simulink model "SiEngineCore"  (R2018a)
settings: Solver=VariableStepAuto  StartTime=0.0  StopTime=inf  RelTol=1e-3  EnableMultiTasking=on
model workspace (MAT data in the model file):
  AFRStoich = 14.6
  AirFilterArea = 0.000962112750162
  AirIntakeVol = 0.0137
  C_eng = 40000
  CompEff = [0.2 0.2 0.2 0.2 0.2 0.2 0.2 0.2 0.2 0.2 0.2 0.2 ... (5000 elements, 50x100)]
  CompMassFlwRate = [4.4091251837e-05 0.00441685548409 0.00879200250921 0.0131688186568 0.0175465480563 0.0219243905675 0.0263014996182 0.0306769799437 0.0350498852261 0.0394192156283 0.0437839152204 0.0481428692931 ... (5000 elements, 50x100)]
  CompPrsRatioBreakPoints = [1 1.02808080808 1.05616161616 1.08424242424 1.11232323232 1.1404040404 1.16848484848 1.19656565657 1.22464646465 1.25272727273 1.28080808081 1.30888888889 1.33696969697 1.36505050505 1.39313131313 1.42121212121 1.44929292929 1.47737373737 1.50545454545 1.53353535354 1.56161616162 1.5896969697 1.61777777778 1.64585858586 1.67393939394 1.70202020202 1.7301010101 1.75818181818 1.78626262626 1.81434343434 1.84242424242 1.87050505051 1.89858585859 1.92666666667 1.95474747475 1.98282828283 2.01090909091 2.03898989899 2.06707070707 2.09515151515 2.12323232323 2.15131313131 2.17939393939 2.20747474747 2.23555555556 2.26363636364 2.29171717172 2.3197979798 2.34787878788 2.37595959596 2.40404040404 2.43212121212 2.4602020202 2.48828282828 2.51636363636 2.54444444444 2.57252525253 2.60060606061 2.62868686869 2.65676767677 2.68484848485 2.71292929293 2.74101010101 2.76909090909 2.79717171717 2.82525252525 2.85333333333 2.88141414141 2.90949494949 2.93757575758 2.96565656566 2.99373737374 3.02181818182 3.0498989899 3.07797979798 3.10606060606 3.13414141414 3.16222222222 3.1903030303 3.21838383838 3.24646464646 3.27454545455 3.30262626263 3.33070707071 3.35878787879 3.38686868687 3.41494949495 3.44303030303 3.47111111111 3.49919191919 3.52727272727 3.55535353535 3.58343434343 3.61151515152 3.6395959596 3.66767676768 3.69575757576 3.72383838384 3.75191919192 3.78]
  CompRefPrs = 101325
  CompRefTemp = 300
  CompSpdBreakPoints = [5 500.713942607 996.427885215 1492.14182782 1987.85577043 2483.56971304 2979.28365564 3474.99759825 3970.71154086 4466.42548347 4962.13942607 5457.85336868 5953.56731129 6449.2812539 6944.9951965 7440.70913911 7936.42308172 8432.13702433 8927.85096693 9423.56490954 9919.27885215 10414.9927948 10910.7067374 11406.42068 11902.1346226 12397.8485652 12893.5625078 13389.2764504 13884.990393 14380.7043356 14876.4182782 15372.1322208 15867.8461634 16363.560106 16859.2740487 17354.9879913 17850.7019339 18346.4158765 18842.1298191 19337.8437617 19833.5577043 20329.2716469 20824.9855895 21320.6995321 21816.4134747 22312.1274173 22807.8413599 23303.5553025 23799.2692452 24294.9831878]
  CoolantTemp = 310
  Cps = 2
  EgrArea = 0.000314159265359
  EgrCoolantTemp = 360
  EgrEffectiveness = 0.8
  ExhSysArea = 0.00138544236023
  ExhSysVol = 0.0044
  IcEffectiveness = 0.7
  InjSlp = 6.45161290323
  LHV = 47300000
  NCyl = 4
  Pstd = 101325
  Rair = 287
  Rexh = 297
  T_cool_start = 355
  T_coolnt_init = 355
  T_coolnt_max = 375
  ThrAngToC = [0  0.001; 90  0.735]
  ThrDiam = 50
  Tstd = 293.15
  TurbEff = [0.1 0.1 0.1 0.1 0.1 0.1 0.1 0.1 0.1 0.1 0.1 0.1 ... (3600 elements, 60x60)]
  TurbMassFlwRate = [0 0 0 0 0 0 0 0 0 0 0 0 ... (3600 elements, 60x60)]
  TurbPrsRatioBreakPoints = [1 1.0066198 1.0187236 1.0343974 1.0529583 1.0740113 1.0972904 1.1226 1.1497884 1.178734 1.2093357 1.2415084 1.2751789 1.3102832 1.346765 1.3845742 1.4236656 1.4639986 1.5055358 1.5482436 1.5920907 1.637048 1.6830889 1.7301885 1.7783234 1.8274719 1.8776134 1.9287287 1.9807996 2.0338087 2.08774 2.142578 2.1983073 2.2549145 2.312386 2.3707092 2.4298713 2.4898612 2.5506673 2.6122787 2.6746855 2.737877 2.801844 2.8665771 2.9320674 2.998306 3.065285 3.1329958 3.201431 3.270583 3.3404438 3.4110072 3.4822657 3.5542126 3.6268415 3.7001462 3.7741203 3.8487577 3.924053 4]
  TurbRefPres = 101325
  TurbRefTemp = 300
  TurbSpdBreakPoints = [0; 236.716179913; 473.432359826; 710.148557878; 946.864755929; 1183.5809177; 1420.29711576; 1657.01327753; 1893.72933048; 2130.44574618; 2367.16179913; 2603.87821484; 2840.59426779; 3077.31050211; 3314.02673644; 3550.74278939; 3787.45884233; 4024.17507666; 4260.89149237; 4497.6077267; 4734.32359826; 4971.04001397; 5207.7562483; 5444.47211987; 5681.18853557; 5917.90495128; 6154.62118561; 6391.33705717; 6628.0532915; 6864.76952583; 7101.48557878; 7338.2018131; 7574.91768467; 7811.6348259; 8048.35015332; 8285.06620627; 8521.78262198; 8758.49885631; 8995.21563477; 9231.93150634; 9468.64755929; 9705.36415637; 9942.08002794; 10178.7958995; 10415.5124966; 10652.2283682; 10888.9442397; 11125.6610182; 11362.3768898; 11599.0927613; 11835.8099026; 12072.52523; 12309.2423712; 12545.9576986; 12782.673933; 13019.3907114; 13256.106583; 13492.8226359; 13729.539233; 13966.2551046]
  TurboInertia = 1.55e-05
  Vd = 0.0015
  Vexh = 0.0016
  Vint = 0.00286
  VolCompOut = 0.0026
  WgArea = 0.000314159265359
  cp_air = 1005
  cp_exh = 1005
  f_co = [6.86026635502e-05 6.86026635502e-05 0.000137130178455 0.000177313004818 0.000153545722458 0.000286109103754 0.00065603982686 0.00012726330728 0.000129286672759 0.000129286672759 0.000129286672759 0.000129286672759 ... (240 elements, 16x15)]
  f_co2 = [0.190124640361 0.190124640361 0.197310430134 0.198841052192 0.19976911847 0.200569885042 0.199664821109 0.20034918367 0.20035007673 0.20035007673 0.20035007673 0.20035007673 ... (240 elements, 16x15)]
  f_del_sa_bpt = [0 0.75 1.5 2.25 3 3.75 4.5 5.25 6 6.75 7.5 8.25 9 9.75 10.5 11.25 12 12.75 13.5 14.25 15 15.75 16.5 17.25 18 18.75 19.5 20.25 21 21.75 22.5 23.25 24 24.75 25.5 26.25 27 27.75 28.5 29.25 30 30.75 31.5 32.25 33 33.75 34.5 35.25 36 36.75 37.5 38.25 39 39.75 40.5 41.25 42 42.75 43.5 44.25 45 45.75 46.5 47.25 48]
  f_exhfrac_n_bpt = [750 1053.57142857 1357.14285714 1660.71428571 1964.28571429 2267.85714286 2571.42857143 2875 3178.57142857 3482.14285714 3785.71428571 4089.28571429 4392.85714286 4696.42857143 5000]
  f_exhfrac_trq_bpt = [0 15 26.4285714286 37.8571428571 49.2857142857 60.7142857143 72.1428571429 83.5714285714 95 106.428571429 117.857142857 129.285714286 140.714285714 152.142857143 163.571428571 175]
  f_fric_temp_bpt = [274 276 278 280 282 284 286 288 290 292 294 296 298 300 302 304 306 308 310 312 314 316 318 320 322 324 326 328 330 332 334 336 338 340 342 344 346 348 350 352 354 356 358 360 362 364 366 368 370 372 374 376 378 380]
  f_fric_temp_mod = [3.96 3.22 2.56 2.26 2.11 2 1.9 1.83 1.76 1.7 1.65 1.6 1.55 1.49 1.44 1.41 1.38 1.35 1.32 1.3 1.27 1.25 1.24 1.21 1.2 1.18 1.16 1.15 1.13 1.12 1.11 1.1 1.09 1.08 1.07 1.06 1.05 1.05 1.04 1.03 1.02 1.02 1.01 1.01 1 1 1 0.999 0.997 0.995 0.993 0.991 0.989 0.987]
  f_hc = [0.00443209119576 0.00443209119576 0.00220684816441 0.00166684424867 0.00138421884093 0.0010658858934 0.00112857643245 0.00117703080332 0.00117597584116 0.00117597584116 0.00117597584116 0.00117597584116 ... (240 elements, 16x15)]
  f_m_lam = [0.94128 0.95565 0.97001 0.98437 0.99008 1.0004 0.97527 0.9549 0.92612 0.89735 0]
  f_m_lam_bpt = [0.65 0.7 0.75 0.8 0.85 0.9 0.95 1 1.05 1.1 2]
  f_m_sa = [1.0019 0.9988 0.9953 0.99173 0.98811 0.98441 0.98065 0.97682 0.97293 0.96897 0.96493 0.96083 0.95666 0.95242 0.94811 0.94373 0.93927 0.93475 0.93015 0.92548 0.92074 0.91592 0.91104 0.90608 0.90105 0.89594 0.89076 0.88551 0.88019 0.8748 0.86933 0.86379 0.85818 0.8525 0.84675 0.84093 0.83503 0.82907 0.82303 0.81693 0.81075 0.80451 0.79819 0.79181 0.78536 0.77884 0.77226 0.7656 0.75888 0.75209 0.74524 0.73832 0.73134 0.72429 0.71717 0.70999 0.70275 0.69682 0.68949 0.68303 0.67548 0.67037 0.66525 0.66014 0.65503]
  f_mdot_air_corr = [1.02156051768 1.00597426471 0.989411677851 1.0033499089 0.984591437857 0.988509040623 1.0326198627 1.02765527362 1.0134784519 0.998280021213 0.981755128787 0.967218261288 ... (400 elements, 20x20)]
  f_mdot_air_corr_ld_bpt = [0.223381333333 0.285105122807 0.346828912281 0.408552701754 0.470276491228 0.532000280702 0.593724070175 0.655447859649 0.717171649123 0.778895438596 0.84061922807 0.902343017544 0.964066807018 1.02579059649 1.08751438596 1.14923817544 1.21096196491 1.27268575439 1.33440954386 1.39613333333]
  f_mdot_air_n_bpt = [750 973.6842 1197.3684 1421.0526 1644.7368 1868.4211 2092.1053 2315.7895 2539.4737 2763.1579 2986.8421 3210.5263 3434.2105 3657.8947 3881.5789 4105.2632 4328.9474 4552.6316 4776.3158 5000]
  f_mdot_intk = [0 0 0 0 0 0 0 0 0 0 0 0 ... (400 elements, 20x20)]
  f_mdot_intk_ecp_bpt = [0 2.6316 5.2632 7.8947 10.5263 13.1579 15.7895 18.4211 21.0526 23.6842 26.3158 28.9474 31.5789 34.2105 36.8421 39.4737 42.1053 44.7368 47.3684 50]
  f_mdot_trpd_bpt = [0 5.7895 11.5789 17.3684 23.1579 28.9474 34.7368 40.5263 46.3158 52.1053 57.8947 63.6842 69.4737 75.2632 81.0526 86.8421 92.6316 98.4211 104.2105 110]
  f_nox = [4.08881357131e-05 4.08881357131e-05 0.00012346903723 0.000189339284589 0.00026637780763 0.000608287545555 0.00102018770254 0.00131576653087 0.00131610412986 0.00131610412986 0.00131610412986 0.00131610412986 ... (240 elements, 16x15)]
  f_nv = [0.64175366561 0.641419295169 0.640125365558 0.638690556197 0.644169906538 0.669178791311 0.731659452876 0.750078238889 0.750078238889 0.750078238889 0.750078238889 0.750078238889 ... (225 elements, 15x15)]
  f_nv_n_bpt = [750 1053.57142857 1357.14285714 1660.71428571 1964.28571429 2267.85714286 2571.42857143 2875 3178.57142857 3482.14285714 3785.71428571 4089.28571429 4392.85714286 4696.42857143 5000]
  f_nv_prs_bpt = [31 40.6428571429 50.2857142857 59.9285714286 69.5714285714 79.2142857143 88.8571428571 98.5 108.142857143 117.785714286 127.428571429 137.071428571 146.714285714 156.357142857 166]
  f_sa_opt = [35.3085 35.3085 21.0105 10.3714 8.5076 7.1426 7.5656 -5.7766 -16.7061 -16.8345 -19.3546 -20.6085 ... (256 elements, 16x16)]
  f_t_exh = [739.936218766 750.584766028 772.770773797 791.235245621 803.106549716 885.862998064 920.498479307 920.498479307 920.498479307 920.498479307 920.498479307 920.498479307 ... (225 elements, 15x15)]
  f_t_exh_l_bpt = [0.2 0.275 0.35 0.425 0.5 0.575 0.65 0.725 0.8 0.875 0.95 1.025 1.1 1.175 1.25]
  f_t_exh_n_bpt = [750 1053.57142857 1357.14285714 1660.71428571 1964.28571429 2267.85714286 2571.42857143 2875 3178.57142857 3482.14285714 3785.71428571 4089.28571429 4392.85714286 4696.42857143 5000]
  f_tm_corr = [0.839360054391 0.833393271885 0.82629554201 0.818442814437 0.811524387436 0.809164184856 0.814606352881 0.826887956871 0.842304598924 0.856886829014 0.869487025783 0.880530414174 ... (400 elements, 20x20)]
  f_tm_corr_n_bpt = [750 973.6842 1197.3684 1421.0526 1644.7368 1868.4211 2092.1053 2315.7895 2539.4737 2763.1579 2986.8421 3210.5263 3434.2105 3657.8947 3881.5789 4105.2632 4328.9474 4552.6316 4776.3158 5000]
  f_tm_corr_nd_bpt = [0.3 0.38947 0.47895 0.56842 0.65789 0.74737 0.83684 0.92632 1.0158 1.1053 1.1947 1.2842 1.3737 1.4632 1.5526 1.6421 1.7316 1.8211 1.9105 2]
  f_tq_fric = [0  4.16  4.8  5.44  6.05  6.64  7.23  7.81  8.39  8.97  9.54  10.1  10.7  11.3  11.9  12.5; 0  4.16  4.8  5.44  6.05  6.64  7.23  7.81  8.39  8.97  9.54  10.1  10.7  11.3  11.9  12.5; 0  4.42  5.07  5.69  6.29  6.89  7.49  8.09  8.69  9.28  9.86  10.4  11  11.6  12.2  12.8; 0  4.69  5.36  5.98  6.58  7.18  7.79  8.41  9.02  9.62  10.2  10.8  11.4  11.9  12.5  13.1; 0  4.88  5.59  6.25  6.87  7.48  8.09  8.71  9.32  9.92  10.5  11.1  11.7  12.3  12.9  13.4; 0  4.94  5.74  6.45  7.12  7.75  8.37  8.99  9.59  10.2  10.8  11.4  11.9  12.6  13.2  13.8; 0  4.93  5.76  6.56  7.29  7.97  8.62  9.23  9.83  10.4  11  11.6  12.2  12.8  13.4  14.1; 0  4.85  5.67  6.57  7.37  8.11  8.8  9.43  10  10.6  11.2  11.8  12.4  13  13.7  14.3; 0  4.74  5.57  6.46  7.34  8.14  8.88  9.55  10.2  10.8  11.4  12  12.6  13.2  13.8  14.4; 0  4.63  5.42  6.27  7.19  8.05  8.83  9.55  10.2  10.9  11.5  12.1  12.7  13.3  14  14.6; 0  4.52  5.29  6.11  6.98  7.84  8.65  9.4  10.1  10.8  11.5  12.1  12.8  13.4  14.1  14.6; 0  4.42  5.18  5.97  6.79  7.6  8.39  9.15  9.88  10.6  11.3  12.1  12.8  13.5  14.1  14.7; 0  4.34  5.09  5.86  6.64  7.42  8.17  8.88  9.6  10.3  11.1  11.9  12.7  13.4  14.1  14.7; 0  4.27  5.01  5.76  6.52  7.28  8.03  8.74  9.39  10.1  10.8  11.6  12.4  13.2  14  14.7; 0  4.21  4.94  5.67  6.42  7.16  7.89  8.59  9.25  9.93  10.7  11.5  12.3  13.1  13.8  14.6; 0  4.15  4.87  5.6  6.33  7.06  7.77  8.47  9.14  9.84  10.6  11.3  12.1  12.9  13.7  14.4]
  f_tq_inr = [25.8508 25.8508 25.8508 25.8508 25.8508 25.8508 25.8508 25.8508 25.8508 25.8508 25.8508 25.8508 ... (256 elements, 16x16)]
  f_tq_inr_l_bpt = [0.1 0.2 0.28571 0.37143 0.45714 0.54286 0.62857 0.71429 0.8 0.88571 0.97143 1.0571 1.1429 1.2286 1.3143 1.4]
  f_tq_inr_n_bpt = [0 750 1053.5714 1357.1429 1660.7143 1964.2857 2267.8571 2571.4286 2875 3178.5714 3482.1429 3785.7143 4089.2857 4392.8571 4696.4286 5000]
  f_tq_nl = [0 15.0012133443 26.4298333923 37.8556656512 49.2846782956 60.7113978793 72.3451969202 77.459652163 78.5324534074 78.5324534074 78.5324534074 78.5324534074 ... (256 elements, 16x16)]
  f_tq_nl_l_bpt = [0 0.2 0.275 0.35 0.425 0.5 0.575 0.65 0.725 0.8 0.875 0.95 1.025 1.1 1.175 1.25]
  f_tq_nl_n_bpt = [0 750 1053.57142857 1357.14285714 1660.71428571 1964.28571429 2267.85714286 2571.42857143 2875 3178.57142857 3482.14285714 3785.71428571 4089.28571429 4392.85714286 4696.42857143 5000]
  f_tq_pump = [0  7.24  7.7  7.82  7.95  8.1  8.27  8.45  8.64  8.78  8.88  8.96  9.03  9.12  9.25  9.45; 0  7.24  7.7  7.82  7.95  8.1  8.27  8.45  8.64  8.78  8.88  8.96  9.03  9.12  9.25  9.45; 0  5.67  6.03  6.37  6.67  6.92  7.14  7.33  7.5  7.67  7.84  8.01  8.19  8.38  8.58  8.8; 0  3.94  4.52  5  5.36  5.6  5.77  5.92  6.1  6.35  6.67  7.02  7.4  7.75  8.06  8.34; 0  2.59  3.14  3.57  3.86  4.05  4.21  4.43  4.76  5.21  5.75  6.32  6.85  7.3  7.65  7.92; 0  1.8  2.25  2.61  2.88  3.11  3.37  3.71  4.17  4.74  5.36  5.96  6.49  6.91  7.23  7.46; 0  1  1.36  1.77  2.15  2.51  2.88  3.31  3.8  4.37  4.98  5.57  6.11  6.57  6.94  7.25; 0  1  1  1  1.09  1.59  2.08  2.6  3.17  3.81  4.49  5.19  5.85  6.44  6.92  7.29; 0  1  1  1  1  1  1.62  2.32  3.05  3.83  4.64  5.44  6.19  6.82  7.31  7.65; 0  1  1  1  1  1  1.35  2.21  3.08  3.97  4.88  5.78  6.64  7.41  8.06  8.58; 0  1  1  1  1  1  1  1.77  2.67  3.58  4.55  5.6  6.73  7.91  9.07  10.1; 0  1  1  1  1  1  1  1.72  2.67  3.61  4.62  5.79  7.15  8.69  10.3  11.9; 0  1  1  1  1  1  1  1.74  2.88  3.96  5.08  6.36  7.86  9.57  11.4  13.2; 0  1  1  1  1  1  1  1.37  2.7  4.01  5.39  6.92  8.65  10.5  12.4  14.2; 0  1  1  1  1  1  1  1.28  2.66  4.14  5.72  7.43  9.28  11.2  13.1  14.8; 0  1  1  1  1  1  1  1.39  2.82  4.39  6.06  7.85  9.73  11.6  13.5  15.1]
  f_vivc = [0.37716 0.38164 0.38611 0.39033 0.39428 0.39795 0.40132 0.40441 0.40719 0.40967 0.41184 0.41372 0.41529 0.41656 0.41755 0.41825 0.41867 0.41884 0.41874 0.41865]
  f_vivc_icp_bpt = [0 2.6316 5.2632 7.8947 10.5263 13.1579 15.7895 18.4211 21.0526 23.6842 26.3158 28.9474 31.5789 34.2105 36.8421 39.4737 42.1053 44.7368 47.3684 50]
  tau_cool = 3000
libraries: autolibfundflw x13, autolibboost x3, simulink x1, autolibcoreeng x1
(part 1 of 2)
settings Model: ModifiedByFormat=The MathWorks, Inc.  Creator=The MathWorks, Inc.  LastModifiedBy=The MathWorks, Inc.
settings DataIOCC: DSMLogging=off
settings CodeAppCC: StateflowObjectComments=on
settings GRTTargetCC: TargetLangStandard=C89/C90 (ANSI)
settings ConfigComp: CovMetricSettings=dsw  CovHtmlReporting=on  CovSaveCumulativeToWorkspaceVar=on  CovSaveSingleToWorkspaceVar=on  CovShowResultsExplorer=off  CovExternalEMLEnable=off
settings SimscapeCC: SimscapeNormalizeSystem=off  SimscapeNominalValues={1, 'bar'; 1, 'cm^3/s'; 1, 'bar*kg/s'; 1, 'kJ/kg'; 1, 'kW'; }

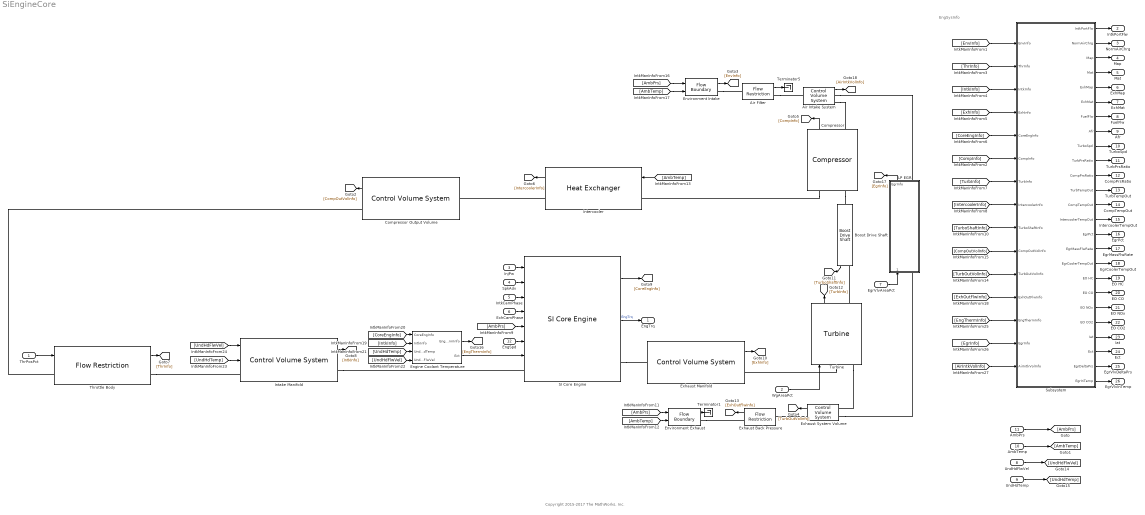
== system SiEngineCore ==
  note: EngSysInfo
  note: Copyright 2015-2017 The MathWorks, Inc.
  ThrPosPct : Inport
  WgAreaPct : Inport  Port=2
  InjPw : Inport  Port=3
  SpkAdv : Inport  Port=4
  IntkCamPhase : Inport  Port=5
  ExhCamPhase : Inport  Port=6
  EgrVlvAreaPct : Inport  Port=7
  UndHdFlwVel : Inport  Port=8
  UndHdTemp : Inport  Port=9
  AmbTemp : Inport  Port=10
  AmbPrs : Inport  Port=11
  EngSpd : Inport  Port=12
  Air Filter : autolibfundflw/Flow Restriction  AreaPopup=Constant  ImageTypePopup=Cold  gamma=cp_air/(cp_air-Rair)  R=Rair  Plim=0.9  Aorf_cnst=AirFilterArea  Cd_cnst=1  Cd_ext=1  Dthr=50  ThrCd=[0.001; 0.735]  ThrAngBpts=[0; 90]
      settings: SourceProductName=Powertrain Blockset  SourceProductBaseCode=PW
  Air Intake System : autolibfundflw/Control Volume System  NumInletPorts=1  NumOutletPorts=2  HeatTransferModelPopup=Constant  ImageTypePopup=Cold  Vch=AirIntakeVol  Pinit=101325  Tinit=298  R=Rair  cp=cp_air  q_he=0  ext_tbl=[40 160 740 2000]  ext_bpts=linspace(0,180,4)  Aext_conv=0.125  m_wall=7  cp_wall=900  Tmass=293.15  Dext_cond=0.004  Aext_cond=0.003  kext=25  Dint_cond=0.004  Aint_cond=0.003  kint=25  int_tbl=[40 160 740 2000]  int_bpts=linspace(0.0020,0.1100,4)  Aint_conv=0.125
      settings: SourceProductName=Powertrain Blockset  SourceProductBaseCode=PW
  Boost Drive Shaft : autolibboost/Boost Drive Shaft  ShaftConfigPopup=Turbocharger  AddTrqTypePopup=No external torque  J_shaft=TurboInertia  w_0=5000*pi/30  w_min=1  w_max=1e6  eta_mech=1
      settings: SourceProductName=Powertrain Blockset  SourceProductBaseCode=PW
  Compressor : autolibboost/Compressor  mdot_corr_tbl=CompMassFlwRate  eta_comp_tbl=CompEff  w_corr_bpts1=CompSpdBreakPoints  Pr_bpts2=CompPrsRatioBreakPoints  T_ref=CompRefTemp  P_ref=CompRefPrs  R=Rair  cp=cp_air
      settings: SourceProductName=Powertrain Blockset  SourceProductBaseCode=PW
  Compressor Output Volume : autolibfundflw/Control Volume System  NumInletPorts=1  NumOutletPorts=1  HeatTransferModelPopup=Constant  ImageTypePopup=Cold  Vch=VolCompOut  Pinit=101325  Tinit=298  R=Rair  cp=cp_air  q_he=0  ext_tbl=[40 160 740 2000]  ext_bpts=linspace(0,180,4)  Aext_conv=0.125  m_wall=7  cp_wall=900  Tmass=293.15  Dext_cond=0.004  Aext_cond=0.003  kext=25  Dint_cond=0.004  Aint_cond=0.003  kint=25  int_tbl=[40 160 740 2000]  int_bpts=linspace(0.0020,0.1100,4)  Aint_conv=0.125
      settings: SourceProductName=Powertrain Blockset  SourceProductBaseCode=PW
  Engine Coolant Temperature : Subsystem
  Environment Exhaust : autolibfundflw/Flow Boundary  PrsTempSrcPopup=External input  ImageTypePopup=Hot  Pcnst=101325  Tcnst=298.15  cp=cp_air
      settings: SourceProductName=Powertrain Blockset  SourceProductBaseCode=PW
  Environment Intake : autolibfundflw/Flow Boundary  PrsTempSrcPopup=External input  ImageTypePopup=Cold  Pcnst=101325  Tcnst=298.15  cp=cp_air
      settings: SourceProductName=Powertrain Blockset  SourceProductBaseCode=PW
  Exhaust Back Pressure : autolibfundflw/Flow Restriction  AreaPopup=Constant  ImageTypePopup=Hot  gamma=cp_exh/(cp_exh-Rexh)  R=Rexh  Plim=0.9  Aorf_cnst=ExhSysArea  Cd_cnst=1  Cd_ext=1  Dthr=50  ThrCd=[0.001; 0.735]  ThrAngBpts=[0; 90]
      settings: SourceProductName=Powertrain Blockset  SourceProductBaseCode=PW
  Exhaust Manifold : autolibfundflw/Control Volume System  NumInletPorts=1  NumOutletPorts=1  HeatTransferModelPopup=Constant  ImageTypePopup=Hot  Vch=Vexh  Pinit=101325  Tinit=298  R=Rexh  cp=cp_exh  q_he=0  ext_tbl=[40 160 740 2000]  ext_bpts=linspace(0,180,4)  Aext_conv=0.125  m_wall=7  cp_wall=900  Tmass=293.15  Dext_cond=0.004  Aext_cond=0.003  kext=25  Dint_cond=0.004  Aint_cond=0.003  kint=25  int_tbl=[40 160 740 2000]  int_bpts=linspace(0.0020,0.1100,4)  Aint_conv=0.125
      settings: SourceProductName=Powertrain Blockset  SourceProductBaseCode=PW
  Exhaust System Volume : autolibfundflw/Control Volume System  NumInletPorts=2  NumOutletPorts=1  HeatTransferModelPopup=Constant  ImageTypePopup=Hot  Vch=ExhSysVol  Pinit=101325  Tinit=298  R=Rexh  cp=cp_exh  q_he=0  ext_tbl=[40 160 740 2000]  ext_bpts=linspace(0,180,4)  Aext_conv=0.125  m_wall=7  cp_wall=900  Tmass=293.15  Dext_cond=0.004  Aext_cond=0.003  kext=25  Dint_cond=0.004  Aint_cond=0.003  kint=25  int_tbl=[40 160 740 2000]  int_bpts=linspace(0.0020,0.1100,4)  Aint_conv=0.125
      settings: SourceProductName=Powertrain Blockset  SourceProductBaseCode=PW
  Intake Manifold : autolibfundflw/Control Volume System  NumInletPorts=1  NumOutletPorts=1  HeatTransferModelPopup=External wall convection  ImageTypePopup=Cold  Vch=Vint  Pinit=101325  Tinit=298  R=Rair  cp=cp_air  q_he=0  ext_tbl=[40 160 740 2000]  ext_bpts=linspace(0,180,4)  Aext_conv=0.125  m_wall=7  cp_wall=900  Tmass=293.15  Dext_cond=0.004  Aext_cond=0.003  kext=25  Dint_cond=0.004  Aint_cond=0.003  kint=25  int_tbl=[40 160 740 2000]  int_bpts=linspace(0.0020,0.1100,4)  Aint_conv=0.125
      settings: SourceProductName=Powertrain Blockset  SourceProductBaseCode=PW
  Intercooler : autolibfundflw/Heat Exchanger  EffctModelPopup=Constant  CoolTempInputPopup=External input  ImageTypePopup=Intercooler  ep_cnst=IcEffectiveness  T_cool_cnst=CoolantTemp  cp=cp_air
      settings: SourceProductName=Powertrain Blockset  SourceProductBaseCode=PW
  LP EGR : Subsystem
  SI Core Engine : autolibcoreeng/SI Core Engine  AirMassFlowOptionPopup=Dual-Independent Variable Cam Phasing  TrqOptionPopup=Torque Structure  NCyl=NCyl  Cps=Cps  Vd=Vd  Rair=Rair  Pstd=Pstd  Tstd=Tstd  f_nv=f_nv  f_nv_prs_bpt=f_nv_prs_bpt  f_nv_n_bpt=f_nv_n_bpt  f_vivc=f_vivc  f_vivc_icp_bpt=f_vivc_icp_bpt  f_tm_corr=f_tm_corr  f_tm_corr_nd_bpt=f_tm_corr_nd_bpt  f_tm_corr_n_bpt=f_tm_corr_n_bpt  f_mdot_intk=f_mdot_intk  f_mdot_intk_ecp_bpt=f_mdot_intk_ecp_bpt  f_mdot_trpd_bpt=f_mdot_trpd_bpt  f_mdot_air_corr=f_mdot_air_corr  f_mdot_air_corr_ld_bpt=f_mdot_air_corr_ld_bpt  f_mdot_air_n_bpt=f_mdot_air_n_bpt  f_tq_nl=f_tq_nl  f_tq_nl_l_bpt=f_tq_nl_l_bpt  f_tq_nl_n_bpt=f_tq_nl_n_bpt  f_tq_inr=f_tq_inr  f_tq_fric=f_tq_fric  f_fric_temp_mod=f_fric_temp_mod  f_fric_temp_bpt=f_fric_temp_bpt  f_tq_pump=f_tq_pump  f_sa_opt=f_sa_opt  f_tq_inr_l_bpt=f_tq_inr_l_bpt  f_tq_inr_n_bpt=f_tq_inr_n_bpt  f_m_sa=f_m_sa  f_del_sa_bpt=f_del_sa_bpt  f_m_lam=f_m_lam  f_m_lam_bpt=f_m_lam_bpt  f_t_exh=f_t_exh  f_t_exh_l_bpt=f_t_exh_l_bpt  f_t_exh_n_bpt=f_t_exh_n_bpt  cp_exh=cp_exh  CO2EmissionsCheckbox=on  COEmissionsCheckbox=on  NOxEmissionsCheckbox=on  HCEmissionsCheckbox=on  PMEmissionsCheckbox=off  f_CO2_frac=f_co2  f_CO_frac=f_co  f_HC_frac=f_hc  f_NOx_frac=f_nox  f_PM_frac=[0 0 0 0 0 0 0 0 0 0 0 0 0 0 0;0 0 0 0 0 0 0 0 0 0 0 0 0 0 0;0 0 0 0 0 0 0 0 0 0 0 0 0 0 0;0 0 0 0 0 0 0 0 0 0 0 0 0 0 0;0 0 0 0 0 0 0 0 0 0 0 0 0 0 0;0 0 0 0 0 0 0 0 0 0 0 0 0 0 0;0 0 0 0 0 0 0 0 0 0 0 0 0 0 0;0 0 0 0 0 0 0 0 0 0 0 0 0 0 0;0 0 0 0 0 0 0 0 0 0 0 0 0 0 0;0 0 0 0 0 0 0 0 0 0 0 0 0 0 0;0 0 0 0 0 0 0 0 0 0 0 0 0 0 0;0 0 0 0 0 0 0 0 0 0 0 0 0 0 0;0 0 0 0 0 0 0 0 0 0 0 0 0 0 0;0 0 0 0 0 0 0 0 0 0 0 0 0 0 0;0 0 0 0 0 0 0 0 0 0 0 0 0 0 0;0 0 0 0 0 0 0 0 0 0 0 0 0 0 0]  f_exhfrac_n_bpt=f_exhfrac_n_bpt  f_exhfrac_trq_bpt=f_exhfrac_trq_bpt  Sinj=InjSlp  afr_stoich=AFRStoich
      settings: SourceProductName=Powertrain Blockset  SourceProductBaseCode=PW
  Subsystem : Subsystem
  Terminator1 : Terminator
  Terminator5 : Terminator
  Throttle Body : autolibfundflw/Flow Restriction  AreaPopup=Throttle body geometry  ImageTypePopup=Cold  gamma=cp_air / (cp_air - Rair)  R=Rair  Plim=0.9  Aorf_cnst=.1  Cd_cnst=1  Cd_ext=1  Dthr=ThrDiam  ThrCd=ThrAngToC(:,2)  ThrAngBpts=ThrAngToC(:,1)
      settings: SourceProductName=Powertrain Blockset  SourceProductBaseCode=PW
  Turbine : autolibboost/Turbine  TurbTypePopup=Fixed geometry  WgIncludeCheckbox=on  mdot_corrfx_tbl=TurbMassFlwRate  mdot_corrvr_tbl=TurbMassFlwRate  eta_turbfx_tbl=TurbEff  eta_turbvr_tbl=TurbEff  w_corrfx_bpts1=TurbSpdBreakPoints  w_corrvr_bpts2=TurbSpdBreakPoints  Pr_fx_bpts2=TurbPrsRatioBreakPoints  Pr_vr_bpts2=TurbPrsRatioBreakPoints  L_rack_bpts3=TurbRackBreakPoints  T_ref=TurbRefTemp  P_ref=TurbRefPres  mdot_thresh=1e-6  A_wgopen=WgArea  Plim_wg=0.95  R=Rexh  cp=cp_exh
      settings: SourceProductName=Powertrain Blockset  SourceProductBaseCode=PW
  EngTrq : Outport
  IntkPortFlw : Outport  Port=2
  NormAirChrg : Outport  Port=3
  Map : Outport  Port=4
  Mat : Outport  Port=5
  ExhMap : Outport  Port=6
  ExhMat : Outport  Port=7
  FuelFlw : Outport  Port=8
  Afr : Outport  Port=9
  TurboSpd : Outport  Port=10
  TurbPrsRatio : Outport  Port=11
  CompPrsRatio : Outport  Port=12
  TurbTempOut : Outport  Port=13
  CompTempOut : Outport  Port=14
  IntercoolerTempOut : Outport  Port=15
  EgrPct : Outport  Port=16
  EgrMassFlwRate : Outport  Port=17
  EgrCoolerTempOut : Outport  Port=18
  EO HC : Outport  Port=19
  EO CO : Outport  Port=20
  EO NOx : Outport  Port=21
  EO CO2 : Outport  Port=22
  Iat : Outport  Port=23
  Ect : Outport  Port=24
  EgrVlvDeltaPrs : Outport  Port=25
  EgrVlvInTemp : Outport  Port=26
  wires:
  Exhaust System Volume/1 -> [TurbOutVolInfo]
  Exhaust Back Pressure/1 -> [ExhOutFlwInfo]
  Environment Intake/1 -> [EnvInfo]
  Air Filter/1 -> Terminator5/1
  Air Intake System/1 -> [AirIntkVolInfo]
  [AmbTemp] -> Intercooler/1
  [AmbTemp] -> Environment Exhaust/2
  [AmbPrs] -> Environment Exhaust/1
  AmbPrs/1 -> [AmbPrs]
  AmbTemp/1 -> [AmbTemp]
  EngSpd/1 -> SI Core Engine/6
  Environment Exhaust/1 -> Terminator1/1
  Compressor Output Volume/1 -> [CompOutVolInfo]
  Intercooler/1 -> [IntercoolerInfo]
  InjPw/1 -> SI Core Engine/1
  SpkAdv/1 -> SI Core Engine/2
  SI Core Engine/2 -> EngTrq/1  "EngTrq"
  Compressor/1 -> [CompInfo]
  Throttle Body/1 -> [ThrInfo]
  Intake Manifold/1 -> [IntkInfo]
  SI Core Engine/1 -> [CoreEngInfo]
  Exhaust Manifold/1 -> [ExhInfo]
  Boost Drive Shaft/1 -> [TurboShaftInfo]
  Turbine/1 -> [TurbInfo]
  WgAreaPct/1 -> Turbine/1
  ThrPosPct/1 -> Throttle Body/1
  [AmbTemp] -> Environment Intake/2
  [AmbPrs] -> Environment Intake/1
  IntkCamPhase/1 -> SI Core Engine/3
  ExhCamPhase/1 -> SI Core Engine/4
  [AmbPrs] -> SI Core Engine/5
  [IntkInfo] -> Engine Coolant Temperature/2(IntkInfo)
  [CoreEngInfo] -> Engine Coolant Temperature/1(CoreEngInfo)
  UndHdFlwVel/1 -> [UndHdFlwVel]
  UndHdTemp/1 -> [UndHdTemp]
  [UndHdTemp] -> Engine Coolant Temperature/3(UndHdTemp)
  [UndHdFlwVel] -> Engine Coolant Temperature/4(UndHdFlwVel)
  [UndHdFlwVel] -> Intake Manifold/1
  [UndHdTemp] -> Intake Manifold/2
  Engine Coolant Temperature/2(Ect) -> SI Core Engine/7
  Engine Coolant Temperature/1(EngThermInfo) -> [EngThermInfo]
  EgrVlvAreaPct/1 -> LP EGR/1(EgrVlvAreaPct)
  LP EGR/1(EgrInfo) -> [EgrInfo]
  Subsystem/2(NormAirChrg) -> NormAirChrg/1
  [EgrInfo] -> Subsystem/14(EgrInfo)
  Subsystem/7(FuelFlw) -> FuelFlw/1
  Subsystem/18(EO HC) -> EO HC/1
  Subsystem/19(EO CO) -> EO CO/1
  [ExhOutFlwInfo] -> Subsystem/12(ExhOutFlwInfo)
  Subsystem/1(IntkPortFlw) -> IntkPortFlw/1
  [IntercoolerInfo] -> Subsystem/8(IntercoolerInfo)
  Subsystem/5(ExhMap) -> ExhMap/1
  [TurboShaftInfo] -> Subsystem/9(TurboShaftInfo)
  [CoreEngInfo] -> Subsystem/5(CoreEngInfo)
  [AirIntkVolInfo] -> Subsystem/15(AirIntkVolInfo)
  [CompInfo] -> Subsystem/6(CompInfo)
  Subsystem/12(TurbTempOut) -> TurbTempOut/1
  [EnvInfo] -> Subsystem/1(EnvInfo)
  [TurbInfo] -> Subsystem/7(TurbInfo)
  Subsystem/3(Map) -> Map/1
  Subsystem/4(Mat) -> Mat/1
  Subsystem/16(EgrMassFlwRate) -> EgrMassFlwRate/1
  [CompOutVolInfo] -> Subsystem/10(CompOutVolInfo)
  [TurbOutVolInfo] -> Subsystem/11(TurbOutVolInfo)
  [IntkInfo] -> Subsystem/3(IntkInfo)
  Subsystem/6(ExhMat) -> ExhMat/1
  Subsystem/15(EgrPct) -> EgrPct/1
  Subsystem/14(IntercoolerTempOut) -> IntercoolerTempOut/1
  Subsystem/22(Iat) -> Iat/1
  Subsystem/9(TurboSpd) -> TurboSpd/1
  Subsystem/8(Afr) -> Afr/1
  Subsystem/23(Ect) -> Ect/1
  Subsystem/11(CompPrsRatio) -> CompPrsRatio/1
  [ThrInfo] -> Subsystem/2(ThrInfo)
  [EngThermInfo] -> Subsystem/13(EngThermInfo)
  Subsystem/17(EgrCoolerTempOut) -> EgrCoolerTempOut/1
  Subsystem/24(EgrDeltaPrs) -> EgrVlvDeltaPrs/1
  Subsystem/21(EO CO2) -> EO CO2/1
  Subsystem/13(CompTempOut) -> CompTempOut/1
  [ExhInfo] -> Subsystem/4(ExhInfo)
  Subsystem/25(EgrInTemp) -> EgrVlvInTemp/1
  Subsystem/10(TurbPrsRatio) -> TurbPrsRatio/1
  Subsystem/20(EO NOx) -> EO NOx/1
  connections:
  Intake Manifold/RConn1 -- SI Core Engine/LConn1
  Throttle Body/RConn1 -- Intake Manifold/LConn1
  Intercooler/RConn1 -- Compressor Output Volume/LConn1
  SI Core Engine/RConn1 -- Exhaust Manifold/LConn1
  Throttle Body/LConn1 -- Compressor Output Volume/RConn1
  Turbine/LConn2 -- Exhaust System Volume/LConn1
  Exhaust Back Pressure/LConn1 -- Exhaust System Volume/RConn1
  Environment Exhaust/RConn1 -- Exhaust Back Pressure/RConn1
  Environment Intake/RConn1 -- Air Filter/LConn1
  Air Filter/RConn1 -- Air Intake System/LConn1
  Compressor/LConn1 -- Intercooler/LConn1
  Compressor/LConn2 -- Boost Drive Shaft/LConn1
  Turbine/RConn1 -- Boost Drive Shaft/RConn1
  Turbine/LConn1 -- Exhaust Manifold/RConn1
  Exhaust System Volume/LConn2 -- LP EGR/LConn1
  Air Intake System/RConn2 -- Compressor/RConn1
  Air Intake System/RConn1 -- LP EGR/RConn1
